simulink model "PortOperationModel"  (R2018b)
settings: Solver=VariableStepAuto  StartTime=0.0  StopTime=20  RelTol=1e-3
values from neighbouring files (symbols this model uses):
  a = 3    [SMC_LV.m]    (also in SlidingModeControl.m)
  b = 3    [SMC_LV.m]    (also in SlidingModeControl.m)
  c = 2    [SMC_LV.m]    (also in SlidingModeControl.m)
  Ini = [1.2; 1.2; 1.2]    [SMC_LV.m]    (also in SlidingModeControl.m)
settings Model: Creator=user  LastModifiedBy=user

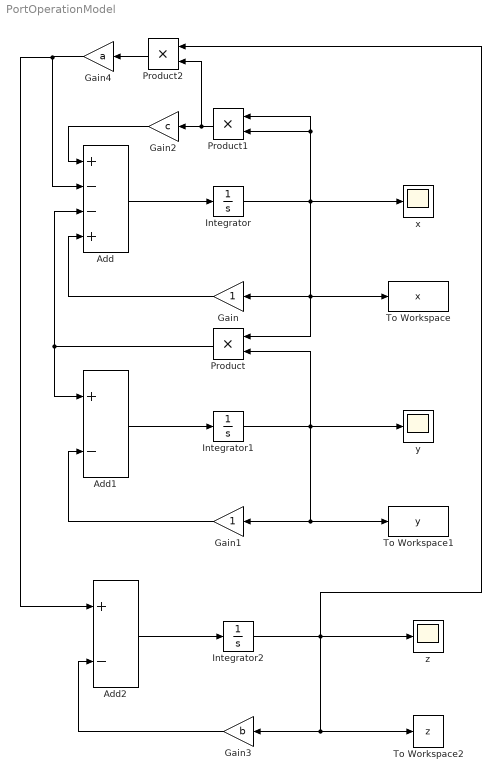
== system PortOperationModel ==
  Add : Sum  Inputs=+--+
  Add1 : Sum  Inputs=+-
  Add2 : Sum  Inputs=+-
  Gain : Gain
  Gain1 : Gain
  Gain2 : Gain  Gain=c
  Gain3 : Gain  Gain=b
  Gain4 : Gain  Gain=a
  Integrator : Integrator  InitialCondition=Ini(1,1)
  Integrator1 : Integrator  InitialCondition=Ini(2,1)
  Integrator2 : Integrator  InitialCondition=Ini(3,1)
  Product : Product
  Product1 : Product
  Product2 : Product
  To Workspace : ToWorkspace  VariableName=x  SampleTime=0.01
  To Workspace1 : ToWorkspace  VariableName=y  SampleTime=0.01
  To Workspace2 : ToWorkspace  VariableName=z  SampleTime=0.01
  x : Scope
  y : Scope
  z : Scope
  wires:
  Add/1 -> Integrator/1
  Integrator/1 -> Product1/1, Product1/2, Product/1, To Workspace/1, Gain/1, x/1
  Gain/1 -> Add/4
  Gain1/1 -> Add1/2
  Integrator1/1 -> Product/2, y/1, Gain1/1, To Workspace1/1
  Add1/1 -> Integrator1/1
  Product/1 -> Add1/1, Add/3
  Product1/1 -> Product2/2, Gain2/1
  Gain2/1 -> Add/1
  Add2/1 -> Integrator2/1
  Integrator2/1 -> z/1, Product2/1, Gain3/1, To Workspace2/1
  Gain3/1 -> Add2/2
  Product2/1 -> Gain4/1
  Gain4/1 -> Add2/1, Add/2
